simulink model "ArmDynamicsOnly"  (R2020a)
settings: Solver=FixedStepAuto  StartTime=0.0  StopTime=tsim  FixedStep=baseRate  MaxStep=0.0001  RelTol=1e-6  AbsTol=1e-6  EnableMultiTasking=on
values from neighbouring files (symbols this model uses):
  b0 = importdata("biases_layer_0.csv")    [Run_Initializer.m]
  b1 = importdata("biases_layer_1.csv")    [Run_Initializer.m]
  b_out = importdata("biases_output.csv")    [Run_Initializer.m]
  baseRate = 0.05    [Run_Initializer.m]
  CHASER_ABSOLUTE_POSITION = true    [Run_Initializer.m]
  drop_states_ARM = [ pi/2, pi/2, 0]    [Run_Initializer.m]
  drop_states_BLACK = [ xLength/2, yLength/2, pi]    [Run_Initializer.m]
  drop_states_BLUE = [ xLength/2, yLength/2, pi]    [Run_Initializer.m]
  drop_states_RED = [ xLength/2+0.5, yLength/2, pi]    [Run_Initializer.m]
  F_Black_X_nominal = 0.2196    [Run_Initializer.m]
  F_Black_Y_nominal = 0.2825    [Run_Initializer.m]
  F_Blue_X_nominal = 0.2196    [Run_Initializer.m]
  F_Blue_Y_nominal = 0.2825    [Run_Initializer.m]
  F_red_X_nominal = 0.2196    [Run_Initializer.m]
  F_red_Y_nominal = 0.2825    [Run_Initializer.m]
  F_thrusters_BLACK = [F_Black_X_nominal; F_Black_X_nominal;                             F_Black_Y_nominal; F_Black_Y_nominal; F_Black_X_nominal;                              F_Black_X_nominal; F_Black_Y_nominal; F_Black_Y_nominal]    [Run_Initializer.m]
  F_thrusters_BLUE = [F_Blue_X_nominal; F_Blue_X_nominal;                             F_Blue_Y_nominal; F_Blue_Y_nominal; F_Blue_X_nominal;                              F_Blue_X_nominal; F_Blue_Y_nominal; F_Blue_Y_nominal]    [Run_Initializer.m]
  F_thrusters_RED = [F_red_X_nominal; F_red_X_nominal;                             F_red_Y_nominal; F_red_Y_nominal; F_red_X_nominal;                              F_red_X_nominal; F_red_Y_nominal; F_red_Y_nominal]    [Run_Initializer.m]
  Gamma1_el = 0.12    [Run_Initializer.m]
  Gamma1_sh = 0.005    [Run_Initializer.m]
  Gamma1_wr = 0.025    [Run_Initializer.m]
  Gamma2_el = 5    [Run_Initializer.m]
  Gamma2_sh = 15    [Run_Initializer.m]
  Gamma2_wr = 5    [Run_Initializer.m]
  Gamma3_el = 10    [Run_Initializer.m]
  Gamma3_sh = 40    [Run_Initializer.m]
  Gamma3_wr = 40    [Run_Initializer.m]
  Gamma4_el = 0.039    [Run_Initializer.m]
  Gamma4_sh = 0.015    [Run_Initializer.m]
  Gamma4_wr = 0.029    [Run_Initializer.m]
  Gamma5_el = 800    [Run_Initializer.m]
  Gamma5_sh = 800    [Run_Initializer.m]
  Gamma5_wr = 800    [Run_Initializer.m]
  Gamma6_el = 0.000001    (= 1e-06)    [Run_Initializer.m]
  Gamma6_sh = 0.005    [Run_Initializer.m]
  Gamma6_wr = 0.02    [Run_Initializer.m]
  HOLD_POINT_RADIUS = 0.95    [Run_Initializer.m]
  home_states_BLACK = [ xLength/2; yLength/2; 0]    [Run_Initializer.m]
  home_states_BLUE = [ xLength/2; yLength/2; 0]    [Run_Initializer.m]
  home_states_RED = [ xLength/2+0.9; yLength/2; pi]    [Run_Initializer.m]
  init_states_BLACK = [ xLength/2; yLength/2; pi]    [Run_Initializer.m]
  init_states_BLUE = [ xLength/2; yLength/2; pi]    [Run_Initializer.m]
  init_states_RED = [ xLength/2+0.9; yLength/2; pi]    [Run_Initializer.m]
  Kd_tb = 1.0    (= 1)    [Run_Initializer.m]
  Kd_tblue = 1    [Run_Initializer.m]
  Kd_tr = 1.0    (= 1)    [Run_Initializer.m]
  Kd_xb = 8    [Run_Initializer.m]
  Kd_xblue = 8    [Run_Initializer.m]
  Kd_xr = 8    [Run_Initializer.m]
  Kd_yb = 8    [Run_Initializer.m]
  Kd_yblue = 8    [Run_Initializer.m]
  Kd_yr = 8    [Run_Initializer.m]
  Kp_tb = 0.1    [Run_Initializer.m]
  Kp_tblue = 0.1    [Run_Initializer.m]
  Kp_tr = 0.1    [Run_Initializer.m]
  Kp_xb = 2    [Run_Initializer.m]
  Kp_xblue = 2    [Run_Initializer.m]
  Kp_xr = 2    [Run_Initializer.m]
  Kp_yb = 2    [Run_Initializer.m]
  Kp_yblue = 2    [Run_Initializer.m]
  Kp_yr = 2    [Run_Initializer.m]
  MAX_BODY_ANGULAR_VELOCITY = 15*180/pi    (= 859.436692696)    [Run_Initializer.m]
  MAX_VELOCITY = 0.1    [Run_Initializer.m]
  noise_variance_BLACK = 0    [Run_Initializer.m]
  noise_variance_BLUE = 0    [Run_Initializer.m]
  noise_variance_RED = 0    [Run_Initializer.m]
  Phase0_End = Phase0_Duration    (= 10)    [Run_Initializer.m]
  Phase1_End = Phase0_Duration + Phase1_Duration    (= 15)    [Run_Initializer.m]
  Phase2_End = Phase0_Duration + Phase1_Duration +                                   Phase2_Duration    (= 45)    [Run_Initializer.m]
  Phase3_End = Phase0_Duration + Phase1_Duration +                                   Phase2_Duration + Phase3_Duration    (= 560)    [Run_Initializer.m]
  Phase3_SubPhase1_End = Phase2_End + Phase3_SubPhase1_Duration    (= 105)    [Run_Initializer.m]
  Phase3_SubPhase2_End = Phase2_End + Phase3_SubPhase1_Duration +                                   Phase3_SubPhase2_Duration    (= 210)    [Run_Initializer.m]
  Phase3_SubPhase3_End = Phase2_End + Phase3_SubPhase1_Duration +                                   Phase3_SubPhase2_Duration +                                  Phase3_SubPhase3_Duration    (= 240)    [Run_Initializer.m]
  Phase3_SubPhase4_End = Phase2_End + Phase3_SubPhase1_Duration +                                   Phase3_SubPhase2_Duration +                                  Phase3_SubPhase3_Duration +                                  Phase3_SubPhase4_Duration    [Run_Initializer.m]
  Phase4_End = Phase0_Duration + Phase1_Duration +                                   Phase2_Duration + Phase3_Duration +                                   Phase4_Duration    (= 680)    [Run_Initializer.m]
  Phase5_End = Phase0_Duration + Phase1_Duration +                                   Phase2_Duration + Phase3_Duration +                                   Phase4_Duration + Phase5_Duration    (= 700)    [Run_Initializer.m]
  relevant_half_range = (upper_state_bound - lower_state_bound)/2    [Run_Initializer.m]
  relevant_state_mean = (lower_state_bound + upper_state_bound)/2    [Run_Initializer.m]
  thruster_dist2CG_BLACK = [72.80;-65.20;61.75;-79.75;65.20;-65.20;74.25;-54.75]    [Run_Initializer.m]
  thruster_dist2CG_BLUE = [83.10;-54.90;71.50;-70.00;54.90;-75.50;64.50;-64.50]    [Run_Initializer.m]
  thruster_dist2CG_RED = [69.38;-56.62;50.01;-81.49;61.12;-68.38;78.99;-52.01]    [Run_Initializer.m]
  w0 = importdata("weights_layer_0.csv")    [Run_Initializer.m]
  w1 = importdata("weights_layer_1.csv")    [Run_Initializer.m]
  w_out = importdata("weights_output.csv")    [Run_Initializer.m]
  xLength = 3.51155    [Run_Initializer.m]
  yLength = 2.41935    [Run_Initializer.m]
undefined symbols (not defined in the file or in its folder): DiscIntNeverNeededParam, model_param, platformSelection, serverRate, simMode
libraries: dspstat3 x18, simulink x11, raspberrypiBasiclib x9, dspsigops x9, embdlinuxlib x7, MainLibrary x4, mspfiltlib x3, dsparch4 x3, etargetslib x1, sensehatlib x1
(part 1 of 14)
settings Model: ExtModeTrigDuration=2  Creator=AlexC  LastModifiedBy=alexa
settings SolverCC: PositivePriorityOrder=on
settings DataIOCC: ReturnWorkspaceOutputs=off
settings OptimizationCC: ZeroExternalMemoryAtStartup=off  ZeroInternalMemoryAtStartup=off  MaxStackSize=64
settings DebuggingCC: MultiTaskDSMMsg=none  ParameterTunabilityLossMsg=error  ArithmeticOperatorsInVariantConditions=warning
settings HardwareCC: ProdBitPerPointer=32  ProdBitPerSizeT=32  ProdBitPerPtrDiffT=32  ProdLargestAtomicInteger=Long  ProdLargestAtomicFloat=Double  ProdWordSize=32  ProdLongLongMode=on  ProdHWDeviceType=ARM Compatible->ARM Cortex
settings SFSimCC: CustomCodeUndefinedFunction=UseInterfaceOnly
settings RTWCC: SystemTargetFile=ert.tlc  HardwareBoard=Raspberry Pi  TemplateMakefile=ert_default_tmf  Toolchain=GNU GCC Raspberry Pi  BuildConfiguration=Faster Runs  TargetLang=C++
settings CodeAppCC: ForceParamTrailComments=on  OperatorAnnotations=on  StateflowObjectComments=on  MATLABSourceComments=on
settings ERTTargetCC: CodeReplacementLibrary=GCC ARM Cortex-A8  ERTCustomFileBanners=off  MatFileLogging=on  SupportContinuousTime=on  SupportNonInlinedSFcns=on  RemoveResetFunc=off  SupportVariableSizeSignals=on  ExtModeTransport=2  ExtModeStaticAlloc=on  ExtModeMexFile=ext_xcp  ExtModeIntrfLevel=Level2 - Open

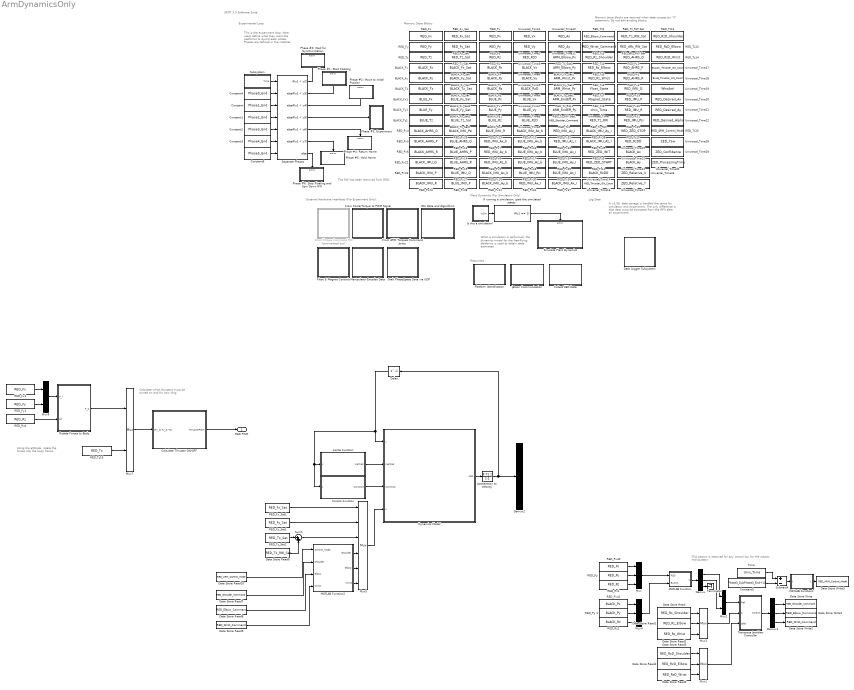
== system ArmDynamicsOnly ==
  note: This is the experiment loop; here, users define what they want the platforms to during each phase. Phases are defined in the intializer.
  note: External Hardware Interfaces (For Experiment Only):
  note: Resources
  note: Plant Dynamics (For Simulation Only)
  note: In v3.08, data storage is handled the same for simulation and experiment. The only difference is that data must be extracted from the RP3 after an experiment.
  note: When a simulation is performed, the dynamics model for the free-flying platforms is used to obtain state estimates.
  note: Memory Store Blocks
  note: SPOT 3.0
      | Software Suite
  note: Experimental Loop
  note: Log Data
  note: Memory store blocks are required when data crosses an "if" statement. Do not edit existing blocks.
  note: The RW has been removed from RED.
  note: This section is reserved for any control law for the robotic manipulator.
  note: Using the attitude, rotate the forces into the body frame.
  note: Calculate which thrusters must be turned on and for how long.
  Acceleration to Velocity : DiscreteIntegrator  IntegratorMethod=Integration: Backward Euler  InitialCondition=[drop_states_RED,drop_states_ARM,0,0,0,0,0,0]  SampleTime=-1  ICPrevOutput=DiscIntNeverNeededParam  ICPrevScaledInput=DiscIntNeverNeededParam
  BLACK_Fx : DataStoreMemory  DataStoreName=BLACK_Fx  ReadBeforeWriteMsg=warning  WriteAfterWriteMsg=warning  WriteAfterReadMsg=warning  ShowAdditionalParam=off
  BLACK_Fx1 : DataStoreMemory  DataStoreName=BLUE_Fx  ReadBeforeWriteMsg=warning  WriteAfterWriteMsg=warning  WriteAfterReadMsg=warning  ShowAdditionalParam=off
  BLACK_Fx_Sat : DataStoreMemory  DataStoreName=BLACK_Fx_Sat  ReadBeforeWriteMsg=warning  WriteAfterWriteMsg=warning  WriteAfterReadMsg=warning  ShowAdditionalParam=off
  BLACK_Fx_Sat1 : DataStoreMemory  DataStoreName=ARM_Elbow_Py  ReadBeforeWriteMsg=warning  WriteAfterWriteMsg=warning  WriteAfterReadMsg=warning  ShowAdditionalParam=off
  BLACK_Fx_Sat2 : DataStoreMemory  DataStoreName=BLUE_Fx_Sat  ReadBeforeWriteMsg=warning  WriteAfterWriteMsg=warning  WriteAfterReadMsg=warning  ShowAdditionalParam=off
  BLACK_Fy : DataStoreMemory  DataStoreName=BLACK_Fy  ReadBeforeWriteMsg=warning  WriteAfterWriteMsg=warning  WriteAfterReadMsg=warning  ShowAdditionalParam=off
  BLACK_Fy1 : DataStoreMemory  DataStoreName=BLUE_Fy  ReadBeforeWriteMsg=warning  WriteAfterWriteMsg=warning  WriteAfterReadMsg=warning  ShowAdditionalParam=off
  BLACK_Fy_Sat : DataStoreMemory  DataStoreName=BLACK_Fy_Sat  ReadBeforeWriteMsg=warning  WriteAfterWriteMsg=warning  WriteAfterReadMsg=warning  ShowAdditionalParam=off
  BLACK_Fy_Sat1 : DataStoreMemory  DataStoreName=ARM_Wrist_Px  ReadBeforeWriteMsg=warning  WriteAfterWriteMsg=warning  WriteAfterReadMsg=warning  ShowAdditionalParam=off
  BLACK_Fy_Sat2 : DataStoreMemory  DataStoreName=BLUE_Fy_Sat  ReadBeforeWriteMsg=warning  WriteAfterWriteMsg=warning  WriteAfterReadMsg=warning  ShowAdditionalParam=off
  BLACK_Px : DataStoreMemory  DataStoreName=BLACK_Px  ReadBeforeWriteMsg=warning  WriteAfterWriteMsg=warning  WriteAfterReadMsg=warning  ShowAdditionalParam=off
  BLACK_Px1 : DataStoreMemory  DataStoreName=BLUE_Px  ReadBeforeWriteMsg=warning  WriteAfterWriteMsg=warning  WriteAfterReadMsg=warning  ShowAdditionalParam=off
  BLACK_Py : DataStoreMemory  DataStoreName=BLACK_Py  ReadBeforeWriteMsg=warning  WriteAfterWriteMsg=warning  WriteAfterReadMsg=warning  ShowAdditionalParam=off
  BLACK_Py1 : DataStoreMemory  DataStoreName=BLUE_Py  ReadBeforeWriteMsg=warning  WriteAfterWriteMsg=warning  WriteAfterReadMsg=warning  ShowAdditionalParam=off
  BLACK_Rz : DataStoreMemory  DataStoreName=BLACK_Rz  ReadBeforeWriteMsg=warning  WriteAfterWriteMsg=warning  WriteAfterReadMsg=warning  ShowAdditionalParam=off
  BLACK_Rz1 : DataStoreMemory  DataStoreName=BLUE_Rz  ReadBeforeWriteMsg=warning  WriteAfterWriteMsg=warning  WriteAfterReadMsg=warning  ShowAdditionalParam=off
  BLACK_Tz : DataStoreMemory  DataStoreName=BLACK_Tz  ReadBeforeWriteMsg=warning  WriteAfterWriteMsg=warning  WriteAfterReadMsg=warning  ShowAdditionalParam=off
  BLACK_Tz1 : DataStoreMemory  DataStoreName=BLUE_Tz  ReadBeforeWriteMsg=warning  WriteAfterWriteMsg=warning  WriteAfterReadMsg=warning  ShowAdditionalParam=off
  BLACK_Tz_Sat : DataStoreMemory  DataStoreName=BLACK_Tz_Sat  ReadBeforeWriteMsg=warning  WriteAfterWriteMsg=warning  WriteAfterReadMsg=warning  ShowAdditionalParam=off
  BLACK_Tz_Sat1 : DataStoreMemory  DataStoreName=ARM_Wrist_Py  ReadBeforeWriteMsg=warning  WriteAfterWriteMsg=warning  WriteAfterReadMsg=warning  ShowAdditionalParam=off
  BLACK_Tz_Sat2 : DataStoreMemory  DataStoreName=BLUE_Tz_Sat  ReadBeforeWriteMsg=warning  WriteAfterWriteMsg=warning  WriteAfterReadMsg=warning  ShowAdditionalParam=off
  Calculate Thruster ON/OFF : Subsystem
  Collect ZED Data : Subsystem
  Constant : Constant  Value=Phase1_End  SampleTime=-1
  Constant1 : Constant  Value=Phase2_End  SampleTime=-1
  Constant2 : Constant  Value=Phase3_End  SampleTime=-1
  Constant3 : Constant  Value=Phase4_End  SampleTime=-1
  Constant4 : Constant  Value=Phase0_End  SampleTime=-1
  Constant5 : Constant  Value=Phase3_SubPhase3_End+10
  Constant6 : Constant  Value=Phase5_End  SampleTime=-1
  Coriolis Function : MATLAB Function  TreatAsAtomicUnit=on
  Data Logger Subsystem : Subsystem
  Data Store Read : DataStoreRead  DataStoreName=RED_Rz_Shoulder
  Data Store Read1 : DataStoreRead  DataStoreName=RED_Rz_Elbow
  Data Store Read10 : DataStoreRead  DataStoreName=RED_ARM_Control_Mode
  Data Store Read2 : DataStoreRead  DataStoreName=RED_Rz_Wrist
  Data Store Read3 : DataStoreRead  DataStoreName=RED_RzD_Shoulder
  Data Store Read4 : DataStoreRead  DataStoreName=RED_RzD_Elbow
  Data Store Read5 : DataStoreRead  DataStoreName=RED_RzD_Wrist
  Data Store Read6 : DataStoreRead  DataStoreName=RED_Tz_RW_Sat
  Data Store Read7 : DataStoreRead  DataStoreName=RED_Shoulder_Command
  Data Store Read8 : DataStoreRead  DataStoreName=RED_Elbow_Command
  Data Store Read9 : DataStoreRead  DataStoreName=RED_Wrist_Command
  Data Store Write : DataStoreWrite  DataStoreName=RED_Shoulder_Command
  Data Store Write1 : DataStoreWrite  DataStoreName=RED_Elbow_Command
  Data Store Write2 : DataStoreWrite  DataStoreName=RED_Wrist_Command
  Data Store Write3 : DataStoreWrite  DataStoreName=RED_ARM_Control_Mode
  Delay : Delay  DelayLength=1
  Demux : Demux  Outputs=3
  Demux1 : Demux  Outputs=3
  Demux2 : Demux  Outputs=12
  Dynamics Model : MATLAB Function  TreatAsAtomicUnit=on
  Float & Magnet Controls : Subsystem
  From ARM Torques Command Joints : Subsystem
  From Force/Torque to PWM Signal : Subsystem  SystemSampleTime=0.1
  From Torque Command RW : Subsystem  Commented=on
  Grab PhaseSpace Data via UDP : Subsystem
  IMU Data and Algorithms : Subsystem
  "If running a simulation, grab the simulated states." : If  IfExpression=u1 == 1  ShowElse=off
  "Inertia Function " : MATLAB Function  TreatAsAtomicUnit=on
  Is this a simulation? : Subsystem
  Jetson Communication : Subsystem
  MATLAB Function : MATLAB Function  TreatAsAtomicUnit=on
  MATLAB Function1 : MATLAB Function  TreatAsAtomicUnit=on
  MATLAB Function2 : MATLAB Function  TreatAsAtomicUnit=on
  Manipulator Encoder Data : Subsystem
  Mux{,1,3..4} (4 alike) : Mux  Inputs=3
  Mux2 : Mux  Inputs=2
  Mux5 : Mux  Inputs=6
  Mux6 : Mux  Inputs=2
  Mux7 : Mux  Inputs=2
  Phase #0: Wait for Synchronization : Subsystem  TreatAsAtomicUnit=on
  "Phase #1: Start Floating " : Subsystem  TreatAsAtomicUnit=on
  Phase #2: Move to Initial Position : Subsystem  TreatAsAtomicUnit=on
  Phase #3: Experiment : Subsystem  TreatAsAtomicUnit=on
  Phase #4: Return Home : Subsystem  TreatAsAtomicUnit=on
  Phase #5: Hold Home : Subsystem  TreatAsAtomicUnit=on
  Phase #6: Stop Floating and Spin Down RW : Subsystem  TreatAsAtomicUnit=on
  Platform Identification : Subsystem
  RED_Fx : DataStoreMemory  DataStoreName=RED_Fx  ReadBeforeWriteMsg=warning  WriteAfterWriteMsg=warning  WriteAfterReadMsg=warning  ShowAdditionalParam=off
  RED_Fx1 : DataStoreRead  DataStoreName=RED_Fx
  RED_Fx_Sat : DataStoreMemory  DataStoreName=RED_Fx_Sat  ReadBeforeWriteMsg=warning  WriteAfterWriteMsg=warning  WriteAfterReadMsg=warning  ShowAdditionalParam=off
  RED_Fx_Sat1 : DataStoreRead  DataStoreName=RED_Fx_Sat
  RED_Fy : DataStoreMemory  DataStoreName=RED_Fy  ReadBeforeWriteMsg=warning  WriteAfterWriteMsg=warning  WriteAfterReadMsg=warning  ShowAdditionalParam=off
  RED_Fy1 : DataStoreRead  DataStoreName=RED_Fy
  RED_Fy_Sat : DataStoreMemory  DataStoreName=RED_Fy_Sat  ReadBeforeWriteMsg=warning  WriteAfterWriteMsg=warning  WriteAfterReadMsg=warning  ShowAdditionalParam=off
  RED_Fy_Sat1 : DataStoreRead  DataStoreName=RED_Fy_Sat
  RED_Px : DataStoreMemory  DataStoreName=RED_Px  ReadBeforeWriteMsg=warning  WriteAfterWriteMsg=warning  WriteAfterReadMsg=warning  ShowAdditionalParam=off
  RED_Px1 : DataStoreMemory  DataStoreName=RED_AHRS_Q  ReadBeforeWriteMsg=warning  WriteAfterWriteMsg=warning  WriteAfterReadMsg=warning  ShowAdditionalParam=off
  RED_Px10 : DataStoreMemory  DataStoreName=BLACK_IMU_Ax_b  ReadBeforeWriteMsg=warning  WriteAfterWriteMsg=warning  WriteAfterReadMsg=warning  ShowAdditionalParam=off
  RED_Px11 : DataStoreMemory  DataStoreName=BLACK_IMU_Ay_b  ReadBeforeWriteMsg=warning  WriteAfterWriteMsg=warning  WriteAfterReadMsg=warning  ShowAdditionalParam=off
  RED_Px12 : DataStoreMemory  DataStoreName=BLACK_IMU_Az_b  ReadBeforeWriteMsg=warning  WriteAfterWriteMsg=warning  WriteAfterReadMsg=warning  ShowAdditionalParam=off
  RED_Px13 : DataStoreMemory  DataStoreName=BLUE_AHRS_Q  ReadBeforeWriteMsg=warning  WriteAfterWriteMsg=warning  WriteAfterReadMsg=warning  ShowAdditionalParam=off
  RED_Px14 : DataStoreMemory  DataStoreName=BLUE_AHRS_P  ReadBeforeWriteMsg=warning  WriteAfterWriteMsg=warning  WriteAfterReadMsg=warning  ShowAdditionalParam=off
  RED_Px15 : DataStoreMemory  DataStoreName=BLUE_AHRS_R  ReadBeforeWriteMsg=warning  WriteAfterWriteMsg=warning  WriteAfterReadMsg=warning  ShowAdditionalParam=off
  RED_Px16 : DataStoreMemory  DataStoreName=BLUE_IMU_Ax_b  ReadBeforeWriteMsg=warning  WriteAfterWriteMsg=warning  WriteAfterReadMsg=warning  ShowAdditionalParam=off
  RED_Px17 : DataStoreMemory  DataStoreName=BLUE_IMU_Ay_b  ReadBeforeWriteMsg=warning  WriteAfterWriteMsg=warning  WriteAfterReadMsg=warning  ShowAdditionalParam=off
  RED_Px18 : DataStoreMemory  DataStoreName=BLUE_IMU_Az_b  ReadBeforeWriteMsg=warning  WriteAfterWriteMsg=warning  WriteAfterReadMsg=warning  ShowAdditionalParam=off
  RED_Px19 : DataStoreMemory  DataStoreName=RED_IMU_Q  ReadBeforeWriteMsg=warning  WriteAfterWriteMsg=warning  WriteAfterReadMsg=warning  ShowAdditionalParam=off
  RED_Px2 : DataStoreMemory  DataStoreName=RED_AHRS_P  ReadBeforeWriteMsg=warning  WriteAfterWriteMsg=warning  WriteAfterReadMsg=warning  ShowAdditionalParam=off
  RED_Px20 : DataStoreMemory  DataStoreName=RED_IMU_P  ReadBeforeWriteMsg=warning  WriteAfterWriteMsg=warning  WriteAfterReadMsg=warning  ShowAdditionalParam=off
  RED_Px21 : DataStoreMemory  DataStoreName=RED_IMU_R  ReadBeforeWriteMsg=warning  WriteAfterWriteMsg=warning  WriteAfterReadMsg=warning  ShowAdditionalParam=off
  RED_Px22 : DataStoreMemory  DataStoreName=BLACK_IMU_Q  ReadBeforeWriteMsg=warning  WriteAfterWriteMsg=warning  WriteAfterReadMsg=warning  ShowAdditionalParam=off
  RED_Px23 : DataStoreMemory  DataStoreName=BLACK_IMU_P  ReadBeforeWriteMsg=warning  WriteAfterWriteMsg=warning  WriteAfterReadMsg=warning  ShowAdditionalParam=off
  RED_Px24 : DataStoreMemory  DataStoreName=BLACK_IMU_R  ReadBeforeWriteMsg=warning  WriteAfterWriteMsg=warning  WriteAfterReadMsg=warning  ShowAdditionalParam=off
  RED_Px25 : DataStoreMemory  DataStoreName=RED_IMU_Psi  ReadBeforeWriteMsg=warning  WriteAfterWriteMsg=warning  WriteAfterReadMsg=warning  ShowAdditionalParam=off
  RED_Px26 : DataStoreMemory  DataStoreName=BLACK_IMU_Psi  ReadBeforeWriteMsg=warning  WriteAfterWriteMsg=warning  WriteAfterReadMsg=warning  ShowAdditionalParam=off
  RED_Px27 : DataStoreMemory  DataStoreName=BLUE_IMU_Q  ReadBeforeWriteMsg=warning  WriteAfterWriteMsg=warning  WriteAfterReadMsg=warning  ShowAdditionalParam=off
  RED_Px28 : DataStoreMemory  DataStoreName=BLUE_IMU_P  ReadBeforeWriteMsg=warning  WriteAfterWriteMsg=warning  WriteAfterReadMsg=warning  ShowAdditionalParam=off
  RED_Px29 : DataStoreMemory  DataStoreName=BLUE_IMU_R  ReadBeforeWriteMsg=warning  WriteAfterWriteMsg=warning  WriteAfterReadMsg=warning  ShowAdditionalParam=off
  RED_Px3 : DataStoreMemory  DataStoreName=RED_AHRS_R  ReadBeforeWriteMsg=warning  WriteAfterWriteMsg=warning  WriteAfterReadMsg=warning  ShowAdditionalParam=off
  RED_Px30 : DataStoreMemory  DataStoreName=BLUE_IMU_Psi  ReadBeforeWriteMsg=warning  WriteAfterWriteMsg=warning  WriteAfterReadMsg=warning  ShowAdditionalParam=off
  RED_Px31 : DataStoreMemory  DataStoreName=RED_IMU_Ax_I  ReadBeforeWriteMsg=warning  WriteAfterWriteMsg=warning  WriteAfterReadMsg=warning  ShowAdditionalParam=off
  RED_Px32 : DataStoreMemory  DataStoreName=RED_IMU_Ay_I  ReadBeforeWriteMsg=warning  WriteAfterWriteMsg=warning  WriteAfterReadMsg=warning  ShowAdditionalParam=off
  RED_Px33 : DataStoreMemory  DataStoreName=RED_IMU_Az_I  ReadBeforeWriteMsg=warning  WriteAfterWriteMsg=warning  WriteAfterReadMsg=warning  ShowAdditionalParam=off
  RED_Px34 : DataStoreMemory  DataStoreName=BLUE_IMU_Ax_I  ReadBeforeWriteMsg=warning  WriteAfterWriteMsg=warning  WriteAfterReadMsg=warning  ShowAdditionalParam=off
  RED_Px35 : DataStoreMemory  DataStoreName=BLUE_IMU_Ay_I  ReadBeforeWriteMsg=warning  WriteAfterWriteMsg=warning  WriteAfterReadMsg=warning  ShowAdditionalParam=off
  RED_Px36 : DataStoreMemory  DataStoreName=BLUE_IMU_Az_I  ReadBeforeWriteMsg=warning  WriteAfterWriteMsg=warning  WriteAfterReadMsg=warning  ShowAdditionalParam=off
  RED_Px37 : DataStoreMemory  DataStoreName=BLACK_IMU_Ax_I  ReadBeforeWriteMsg=warning  WriteAfterWriteMsg=warning  WriteAfterReadMsg=warning  ShowAdditionalParam=off
  RED_Px38 : DataStoreMemory  DataStoreName=BLACK_IMU_Ay_I  ReadBeforeWriteMsg=warning  WriteAfterWriteMsg=warning  WriteAfterReadMsg=warning  ShowAdditionalParam=off
  RED_Px39 : DataStoreMemory  DataStoreName=BLACK_IMU_Az_I  ReadBeforeWriteMsg=warning  WriteAfterWriteMsg=warning  WriteAfterReadMsg=warning  ShowAdditionalParam=off
  RED_Px4 : DataStoreMemory  DataStoreName=BLACK_AHRS_Q  ReadBeforeWriteMsg=warning  WriteAfterWriteMsg=warning  WriteAfterReadMsg=warning  ShowAdditionalParam=off
  RED_Px40 : DataStoreRead  DataStoreName=RED_Px
  RED_Px41 : DataStoreRead  DataStoreName=BLACK_Px
  RED_Px5 : DataStoreMemory  DataStoreName=BLACK_AHRS_P  ReadBeforeWriteMsg=warning  WriteAfterWriteMsg=warning  WriteAfterReadMsg=warning  ShowAdditionalParam=off
  RED_Px6 : DataStoreMemory  DataStoreName=BLACK_AHRS_R  ReadBeforeWriteMsg=warning  WriteAfterWriteMsg=warning  WriteAfterReadMsg=warning  ShowAdditionalParam=off
  RED_Px7 : DataStoreMemory  DataStoreName=RED_IMU_Ax_b  ReadBeforeWriteMsg=warning  WriteAfterWriteMsg=warning  WriteAfterReadMsg=warning  ShowAdditionalParam=off
  RED_Px8 : DataStoreMemory  DataStoreName=RED_IMU_Ay_b  ReadBeforeWriteMsg=warning  WriteAfterWriteMsg=warning  WriteAfterReadMsg=warning  ShowAdditionalParam=off
  RED_Px9 : DataStoreMemory  DataStoreName=RED_IMU_Az_b  ReadBeforeWriteMsg=warning  WriteAfterWriteMsg=warning  WriteAfterReadMsg=warning  ShowAdditionalParam=off
  RED_Py : DataStoreMemory  DataStoreName=RED_Py  ReadBeforeWriteMsg=warning  WriteAfterWriteMsg=warning  WriteAfterReadMsg=warning  ShowAdditionalParam=off
  "RED_Py " : DataStoreRead  DataStoreName=RED_Py
  RED_Py 1 : DataStoreRead  DataStoreName=BLACK_Py
  RED_Rz : DataStoreMemory  DataStoreName=RED_Rz  ReadBeforeWriteMsg=warning  WriteAfterWriteMsg=warning  WriteAfterReadMsg=warning  ShowAdditionalParam=off
  RED_Rz1 : DataStoreRead  DataStoreName=RED_Rz
  RED_Rz2 : DataStoreRead  DataStoreName=BLACK_Rz
  RED_Rz4 : DataStoreRead  DataStoreName=RED_Rz
  RED_Tz : DataStoreMemory  DataStoreName=RED_Tz  ReadBeforeWriteMsg=warning  WriteAfterWriteMsg=warning  WriteAfterReadMsg=warning  ShowAdditionalParam=off
  RED_Tz1 : DataStoreMemory  DataStoreName=RED_Shoulder_Command  ReadBeforeWriteMsg=warning  WriteAfterWriteMsg=warning  WriteAfterReadMsg=warning  ShowAdditionalParam=off
  RED_Tz10 : DataStoreMemory  DataStoreName=RED_ZED_STOP  ReadBeforeWriteMsg=warning  WriteAfterWriteMsg=warning  WriteAfterReadMsg=warning  ShowAdditionalParam=off
  RED_Tz11 : DataStoreMemory  DataStoreName=RED_ZED_START  ReadBeforeWriteMsg=warning  WriteAfterWriteMsg=warning  WriteAfterReadMsg=warning  ShowAdditionalParam=off
  RED_Tz12 : DataStoreMemory  DataStoreName=RED_RzD_Shoulder  ReadBeforeWriteMsg=warning  WriteAfterWriteMsg=warning  WriteAfterReadMsg=warning  ShowAdditionalParam=off
  RED_Tz13 : DataStoreMemory  DataStoreName=RED_RzD_Elbow  ReadBeforeWriteMsg=warning  WriteAfterWriteMsg=warning  WriteAfterReadMsg=warning  ShowAdditionalParam=off
  RED_Tz14 : DataStoreMemory  DataStoreName=RED_RzD_Wrist  ReadBeforeWriteMsg=warning  WriteAfterWriteMsg=warning  WriteAfterReadMsg=warning  ShowAdditionalParam=off
  RED_Tz15 : DataStoreMemory  DataStoreName=RED_ARM_Control_Mode  ReadBeforeWriteMsg=warning  WriteAfterWriteMsg=warning  WriteAfterReadMsg=warning  ShowAdditionalParam=off
  RED_Tz16 : DataStoreRead  DataStoreName=RED_Tz
  RED_Tz2 : DataStoreMemory  DataStoreName=RED_Elbow_Command  ReadBeforeWriteMsg=warning  WriteAfterWriteMsg=warning  WriteAfterReadMsg=warning  ShowAdditionalParam=off
  RED_Tz3 : DataStoreMemory  DataStoreName=RED_Wrist_Command  ReadBeforeWriteMsg=warning  WriteAfterWriteMsg=warning  WriteAfterReadMsg=warning  ShowAdditionalParam=off
  RED_Tz4 : DataStoreMemory  DataStoreName=RED_Rz_Shoulder  ReadBeforeWriteMsg=warning  WriteAfterWriteMsg=warning  WriteAfterReadMsg=warning  ShowAdditionalParam=off
  RED_Tz5 : DataStoreMemory  DataStoreName=RED_Rz_Elbow  ReadBeforeWriteMsg=warning  WriteAfterWriteMsg=warning  WriteAfterReadMsg=warning  ShowAdditionalParam=off
  RED_Tz6 : DataStoreMemory  DataStoreName=RED_Rz_Wrist  ReadBeforeWriteMsg=warning  WriteAfterWriteMsg=warning  WriteAfterReadMsg=warning  ShowAdditionalParam=off
  RED_Tz7 : DataStoreMemory  DataStoreName=Float_State  ReadBeforeWriteMsg=warning  WriteAfterWriteMsg=warning  WriteAfterReadMsg=warning  ShowAdditionalParam=off
  RED_Tz8 : DataStoreMemory  DataStoreName=Magnet_State  ReadBeforeWriteMsg=warning  WriteAfterWriteMsg=warning  WriteAfterReadMsg=warning  ShowAdditionalParam=off
  RED_Tz9 : DataStoreMemory  DataStoreName=RED_ZED_INIT  ReadBeforeWriteMsg=warning  WriteAfterWriteMsg=warning  WriteAfterReadMsg=warning  ShowAdditionalParam=off
  RED_Tz_RW : DataStoreMemory  DataStoreName=RED_Tz_RW  ReadBeforeWriteMsg=warning  WriteAfterWriteMsg=warning  WriteAfterReadMsg=warning  ShowAdditionalParam=off
  RED_Tz_RW Sat : DataStoreMemory  DataStoreName=RED_Tz_RW_Sat  ReadBeforeWriteMsg=warning  WriteAfterWriteMsg=warning  WriteAfterReadMsg=warning  ShowAdditionalParam=off
  RED_Tz_RW Sat1 : DataStoreMemory  DataStoreName=ARM_EndEff_Py  ReadBeforeWriteMsg=warning  WriteAfterWriteMsg=warning  WriteAfterReadMsg=warning  ShowAdditionalParam=off
  RED_Tz_RW1 : DataStoreMemory  DataStoreName=ARM_EndEff_Px  ReadBeforeWriteMsg=warning  WriteAfterWriteMsg=warning  WriteAfterReadMsg=warning  ShowAdditionalParam=off
  RED_Tz_Sat : DataStoreMemory  DataStoreName=RED_Tz_Sat  ReadBeforeWriteMsg=warning  WriteAfterWriteMsg=warning  WriteAfterReadMsg=warning  ShowAdditionalParam=off
  RED_Tz_Sat1 : DataStoreMemory  DataStoreName=ARM_Elbow_Px  ReadBeforeWriteMsg=warning  WriteAfterWriteMsg=warning  WriteAfterReadMsg=warning  ShowAdditionalParam=off
  RED_Tz_Sat2 : DataStoreRead  DataStoreName=RED_Tz_Sat
  RED_dRz_RW Sat : DataStoreMemory  DataStoreName=RED_dRz_RW_Sat  ReadBeforeWriteMsg=warning  WriteAfterWriteMsg=warning  WriteAfterReadMsg=warning  ShowAdditionalParam=off
  Rotate Forces to Body : Subsystem
  Separate Phases : If  NumInputs=7  IfExpression=u1 < u2  ElseIfExpressions=u1 < u3, u1 < u4, u1 < u5, u1 < u6, u1 < u7
  Simulate Plant Dynamics : Subsystem  TreatAsAtomicUnit=on
  Subsystem : Subsystem
  Subtract4 : Sum  Inputs=+-
  Sum1 : Sum  Inputs=|++
  Terminator : Terminator
  Time : DataStoreRead  DataStoreName=Univ_Time
  Transpose Jacobian Controller : Subsystem
  Universal_Time : DataStoreMemory  DataStoreName=Univ_Time  ReadBeforeWriteMsg=warning  WriteAfterWriteMsg=warning  WriteAfterReadMsg=warning  ShowAdditionalParam=off
  Universal_Time1 : DataStoreMemory  DataStoreName=RED_Vx  ReadBeforeWriteMsg=warning  WriteAfterWriteMsg=warning  WriteAfterReadMsg=warning  ShowAdditionalParam=off
  Universal_Time10 : DataStoreMemory  DataStoreName=RED_Ax  ReadBeforeWriteMsg=warning  WriteAfterWriteMsg=warning  WriteAfterReadMsg=warning  ShowAdditionalParam=off
  Universal_Time11 : DataStoreMemory  DataStoreName=RED_Ay  ReadBeforeWriteMsg=warning  WriteAfterWriteMsg=warning  WriteAfterReadMsg=warning  ShowAdditionalParam=off
  Universal_Time12 : DataStoreMemory  DataStoreName=BLACK_Ax  ReadBeforeWriteMsg=warning  WriteAfterWriteMsg=warning  WriteAfterReadMsg=warning  ShowAdditionalParam=off
  Universal_Time13 : DataStoreMemory  DataStoreName=BLACK_Ay  ReadBeforeWriteMsg=warning  WriteAfterWriteMsg=warning  WriteAfterReadMsg=warning  ShowAdditionalParam=off
  Universal_Time14 : DataStoreMemory  DataStoreName=BLACK_RzDD  ReadBeforeWriteMsg=warning  WriteAfterWriteMsg=warning  WriteAfterReadMsg=warning  ShowAdditionalParam=off
  Universal_Time15 : DataStoreMemory  DataStoreName=RED_RzDD  ReadBeforeWriteMsg=warning  WriteAfterWriteMsg=warning  WriteAfterReadMsg=warning  ShowAdditionalParam=off
  Universal_Time16 : DataStoreMemory  DataStoreName=RED_Thruster_ON_Count  ReadBeforeWriteMsg=warning  WriteAfterWriteMsg=warning  WriteAfterReadMsg=warning  ShowAdditionalParam=off
  Universal_Time17 : DataStoreMemory  DataStoreName=BLACK_Thruster_ON_Count  ReadBeforeWriteMsg=warning  WriteAfterWriteMsg=warning  WriteAfterReadMsg=warning  ShowAdditionalParam=off
  Universal_Time18 : DataStoreMemory  DataStoreName=BLUE_Thruster_ON_Count  ReadBeforeWriteMsg=warning  WriteAfterWriteMsg=warning  WriteAfterReadMsg=warning  ShowAdditionalParam=off
  Universal_Time19 : DataStoreMemory  DataStoreName=WhoAmI  ReadBeforeWriteMsg=warning  WriteAfterWriteMsg=warning  WriteAfterReadMsg=warning  ShowAdditionalParam=off
  Universal_Time2 : DataStoreMemory  DataStoreName=RED_Vy  ReadBeforeWriteMsg=warning  WriteAfterWriteMsg=warning  WriteAfterReadMsg=warning  ShowAdditionalParam=off
  Universal_Time20 : DataStoreMemory  DataStoreName=RED_Desired_Ax  ReadBeforeWriteMsg=warning  WriteAfterWriteMsg=warning  WriteAfterReadMsg=warning  ShowAdditionalParam=off
  Universal_Time21 : DataStoreMemory  DataStoreName=RED_Desired_Ay  ReadBeforeWriteMsg=warning  WriteAfterWriteMsg=warning  WriteAfterReadMsg=warning  ShowAdditionalParam=off
  Universal_Time22 : DataStoreMemory  DataStoreName=RED_Desired_Alpha  ReadBeforeWriteMsg=warning  WriteAfterWriteMsg=warning  WriteAfterReadMsg=warning  ShowAdditionalParam=off
  Universal_Time26 : DataStoreMemory  DataStoreName=ZED_Relative_X  ReadBeforeWriteMsg=warning  WriteAfterWriteMsg=warning  WriteAfterReadMsg=warning  ShowAdditionalParam=off
  Universal_Time27 : DataStoreMemory  DataStoreName=ZED_Relative_Y  ReadBeforeWriteMsg=warning  WriteAfterWriteMsg=warning  WriteAfterReadMsg=warning  ShowAdditionalParam=off
  Universal_Time28 : DataStoreMemory  DataStoreName=ZED_Yaw  ReadBeforeWriteMsg=warning  WriteAfterWriteMsg=warning  WriteAfterReadMsg=warning  ShowAdditionalParam=off
  Universal_Time29 : DataStoreMemory  DataStoreName=ZED_Confidence  ReadBeforeWriteMsg=warning  WriteAfterWriteMsg=warning  WriteAfterReadMsg=warning  ShowAdditionalParam=off
  Universal_Time3 : DataStoreMemory  DataStoreName=RED_RzD  ReadBeforeWriteMsg=warning  WriteAfterWriteMsg=warning  WriteAfterReadMsg=warning  ShowAdditionalParam=off
  Universal_Time30 : DataStoreMemory  DataStoreName=ZED_ProcessingTime  ReadBeforeWriteMsg=warning  WriteAfterWriteMsg=warning  WriteAfterReadMsg=warning  ShowAdditionalParam=off
  Universal_Time4 : DataStoreMemory  DataStoreName=BLACK_Vx  ReadBeforeWriteMsg=warning  WriteAfterWriteMsg=warning  WriteAfterReadMsg=warning  ShowAdditionalParam=off
  Universal_Time5 : DataStoreMemory  DataStoreName=BLACK_Vy  ReadBeforeWriteMsg=warning  WriteAfterWriteMsg=warning  WriteAfterReadMsg=warning  ShowAdditionalParam=off
  Universal_Time6 : DataStoreMemory  DataStoreName=BLACK_RzD  ReadBeforeWriteMsg=warning  WriteAfterWriteMsg=warning  WriteAfterReadMsg=warning  ShowAdditionalParam=off
  Universal_Time7 : DataStoreMemory  DataStoreName=BLUE_Vx  ReadBeforeWriteMsg=warning  WriteAfterWriteMsg=warning  WriteAfterReadMsg=warning  ShowAdditionalParam=off
  Universal_Time8 : DataStoreMemory  DataStoreName=BLUE_Vy  ReadBeforeWriteMsg=warning  WriteAfterWriteMsg=warning  WriteAfterReadMsg=warning  ShowAdditionalParam=off
  Universal_Time9 : DataStoreMemory  DataStoreName=BLUE_RzD  ReadBeforeWriteMsg=warning  WriteAfterWriteMsg=warning  WriteAfterReadMsg=warning  ShowAdditionalParam=off
  RED PWM : Outport  VectorParamsAs1DForOutWhenUnconnected=off
  wires:
  "If running a simulation, grab the simulated states."/1 -> Simulate Plant Dynamics/Action
  Separate Phases/3 -> Phase #2: Move to Initial Position/Action
  Constant1/1 -> Separate Phases/4
  Constant/1 -> Separate Phases/3
  Subsystem/1(Time) -> Separate Phases/1
  Separate Phases/1 -> Phase #0: Wait for Synchronization/Action
  Is this a simulation?/1(isSim) -> "If running a simulation, grab the simulated states."/1
  Constant2/1 -> Separate Phases/5
  Separate Phases/2 -> "Phase #1: Start Floating "/Action
  Separate Phases/6 -> Phase #5: Hold Home/Action
  Separate Phases/5 -> Phase #4: Return Home/Action
  Separate Phases/4 -> Phase #3: Experiment/Action
  Separate Phases/7 -> Phase #6: Stop Floating and Spin Down RW/Action
  Constant6/1 -> Separate Phases/7
  Constant4/1 -> Separate Phases/2
  Constant3/1 -> Separate Phases/6
  Demux/1 -> Mux2/1
  Mux/1 -> MATLAB Function/1(RED)
  RED_Px41/1 -> Mux4/1
  Mux2/1 -> Transpose Jacobian Controller/1(Ref)
  Subtract4/1 -> MATLAB Function1/1(Sim_Time)
  Mux4/1 -> MATLAB Function/2(BLACK)
  "RED_Py "/1 -> Mux/2
  Time/1 -> Subtract4/1
  Constant5/1 -> Subtract4/2
  Data Store Read5/1 -> Mux1/3
  RED_Py 1/1 -> Mux4/2
  RED_Rz1/1 -> Mux/3
  Demux/3 -> Terminator/1
  Mux1/1 -> Transpose Jacobian Controller/3(qdot)
  Data Store Read3/1 -> Mux1/1
  Mux3/1 -> Transpose Jacobian Controller/2(q)
  RED_Rz2/1 -> Mux4/3
  Data Store Read2/1 -> Mux3/3
  Demux1/2 -> Data Store Write1/1
  Data Store Read/1 -> Mux3/1
  Transpose Jacobian Controller/1(Control) -> Demux1/1
  Demux1/3 -> Data Store Write2/1
  Data Store Read1/1 -> Mux3/2
  MATLAB Function/1(p_red_target) -> Demux/1
  MATLAB Function1/1(Control_Mode) -> Data Store Write3/1
  Data Store Read4/1 -> Mux1/2
  Demux1/1 -> Data Store Write/1
  RED_Px40/1 -> Mux/1
  Demux/2 -> Mux2/2
  Data Store Read8/1 -> MATLAB Function2/3("Elbow ")
  Data Store Read9/1 -> MATLAB Function2/4("Wrist ")
  Data Store Read10/1 -> MATLAB Function2/1(Control_Mode)
  Coriolis Function/1(CoriolisS) -> Dynamics Model/3(CoriolisS)
  RED_Fy_Sat1/1 -> Mux5/2
  Dynamics Model/1(xdot) -> Acceleration to Velocity/1
  "Inertia Function "/1(InertiaS) -> Dynamics Model/2(InertiaS)
  Acceleration to Velocity/1 -> Delay/1, Demux2/1
  MATLAB Function2/1(Shoulder) -> Mux5/4
  MATLAB Function2/2(Elbow) -> Mux5/5
  Data Store Read6/1 -> Sum1/2
  MATLAB Function2/3(Wrist) -> Mux5/6
  Data Store Read7/1 -> MATLAB Function2/2("Shoulder ")
  RED_Fx_Sat1/1 -> Mux5/1
  Sum1/1 -> Mux5/3
  Delay/1 -> Coriolis Function/1(x), "Inertia Function "/1(x), Dynamics Model/1(x)
  RED_Tz_Sat2/1 -> Sum1/1
  Mux5/1 -> Dynamics Model/4(u)
  Calculate Thruster ON/OFF/1(ThrusterPWM) -> RED PWM/1
  Rotate Forces to Body/1(F_b) -> Mux7/1
  RED_Fx1/1 -> Mux6/1
  Mux7/1 -> Calculate Thruster ON/OFF/1("[Fx_b; Fy_b; Tz]")
  RED_Tz16/1 -> Mux7/2
  RED_Fy1/1 -> Mux6/2
  RED_Rz4/1 -> Rotate Forces to Body/2(Rz)
  Mux6/1 -> Rotate Forces to Body/1("F_I ")

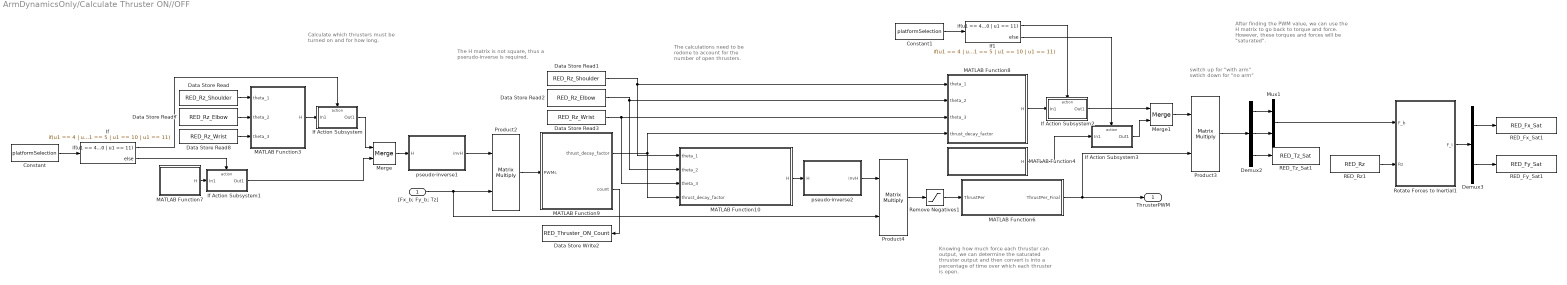
== system ArmDynamicsOnly/Calculate Thruster ON//OFF ==
  note: switch up for "with arm"
      | swtich down for "no arm"
  note: Knowing how much force each thruster can output, we can determine the saturated thruster output and then convert is into a percentage of time over which each thruster is open.
  note: The H matrix is not square, thus a pserudo-inverse is required.
  note: After finding the PWM value, we can use the H matrix to go back to torque and force. However, these torques and forces will be "saturated".
  note: Calculate which thrusters must be turned on and for how long.
  note: The calculations need to be redone to account for the number of open thrusters.
  "[Fx_b; Fy_b; Tz]" : Inport
  Constant : Constant  Value=platformSelection
  Constant1 : Constant  Value=platformSelection
  Data Store Read : DataStoreRead  DataStoreName=RED_Rz_Shoulder
  Data Store Read1 : DataStoreRead  DataStoreName=RED_Rz_Shoulder
  Data Store Read2 : DataStoreRead  DataStoreName=RED_Rz_Elbow
  Data Store Read3 : DataStoreRead  DataStoreName=RED_Rz_Wrist
  Data Store Read7 : DataStoreRead  DataStoreName=RED_Rz_Elbow
  Data Store Read8 : DataStoreRead  DataStoreName=RED_Rz_Wrist
  Data Store Write2 : DataStoreWrite  DataStoreName=RED_Thruster_ON_Count
  Demux2 : Demux  Outputs=3
  Demux3 : Demux  Outputs=2
  If : If  IfExpression=u1 == 4 | u1 == 5 | u1 == 10 | u1 == 11
  If Action Subsystem : Subsystem  TreatAsAtomicUnit=on
  If Action Subsystem1 : Subsystem  TreatAsAtomicUnit=on
  If Action Subsystem2 : Subsystem  TreatAsAtomicUnit=on
  If Action Subsystem3 : Subsystem  TreatAsAtomicUnit=on
  If1 : If  IfExpression=u1 == 4 | u1 == 5 | u1 == 10 | u1 == 11
  MATLAB Function10 : MATLAB Function  TreatAsAtomicUnit=on
  MATLAB Function3 : MATLAB Function  TreatAsAtomicUnit=on
  MATLAB Function4 : MATLAB Function  TreatAsAtomicUnit=on
  MATLAB Function6 : MATLAB Function  TreatAsAtomicUnit=on
  MATLAB Function7 : MATLAB Function  TreatAsAtomicUnit=on
  MATLAB Function8 : MATLAB Function  TreatAsAtomicUnit=on
  MATLAB Function9 : MATLAB Function  TreatAsAtomicUnit=on
  Merge : Merge
  Merge1 : Merge
  Mux1 : Mux  Inputs=2
  Product2 : Product  Multiplication=Matrix(*)
  Product3 : Product  Multiplication=Matrix(*)
  Product4 : Product  Multiplication=Matrix(*)
  RED_Fx_Sat1 : DataStoreWrite  DataStoreName=RED_Fx_Sat
  RED_Fy_Sat1 : DataStoreWrite  DataStoreName=RED_Fy_Sat
  RED_Rz1 : DataStoreRead  DataStoreName=RED_Rz
  RED_Tz_Sat1 : DataStoreWrite  DataStoreName=RED_Tz_Sat
  Remove Negatives1 : Saturate  UpperLimit=1000  LowerLimit=0
  Rotate Forces to Inertial1 : Subsystem
  pseudo-inverse1 : Subsystem
  pseudo-inverse2 : Subsystem
  ThrusterPWM : Outport  VectorParamsAs1DForOutWhenUnconnected=off
  wires:
  MATLAB Function7/1(H) -> If Action Subsystem1/1(In1)
  If Action Subsystem3/1(Out1) -> Merge1/2
  Demux2/3 -> RED_Tz_Sat1/1
  Product3/1 -> Demux2/1
  Data Store Read8/1 -> MATLAB Function3/3(theta_3)
  Data Store Read2/1 -> MATLAB Function8/2(theta_2), MATLAB Function10/2(theta_2)
  MATLAB Function8/1(H) -> If Action Subsystem2/1(In1)
  Data Store Read/1 -> MATLAB Function3/1(theta_1)
  If1/2 -> If Action Subsystem3/Action
  Demux3/2 -> RED_Fy_Sat1/1
  MATLAB Function9/2(count) -> Data Store Write2/1
  If Action Subsystem/1(Out1) -> Merge/1
  MATLAB Function3/1(H) -> If Action Subsystem/1(In1)
  RED_Rz1/1 -> Rotate Forces to Inertial1/2(Rz)
  Data Store Read3/1 -> MATLAB Function8/3(theta_3), MATLAB Function10/3(theta_3)
  MATLAB Function4/1(H) -> If Action Subsystem3/1(In1)
  Demux3/1 -> RED_Fx_Sat1/1
  pseudo-inverse1/1(invH) -> Product2/1
  MATLAB Function6/1(ThrustPer_Final) -> ThrusterPWM/1, Product3/2
  If Action Subsystem1/1(Out1) -> Merge/2
  Demux2/2 -> Mux1/2
  Constant1/1 -> If1/1
  If Action Subsystem2/1(Out1) -> Merge1/1
  Demux2/1 -> Mux1/1
  "[Fx_b; Fy_b; Tz]"/1 -> Product4/2, Product2/2
  MATLAB Function9/1(thrust_decay_factor) -> MATLAB Function10/4(thrust_decay_factor), MATLAB Function8/4(thrust_decay_factor)
  If/2 -> If Action Subsystem1/Action
  Mux1/1 -> Rotate Forces to Inertial1/1("F_b ")
  Product2/1 -> MATLAB Function9/1(PWMs)
  Product4/1 -> Remove Negatives1/1
  Rotate Forces to Inertial1/1(F_I) -> Demux3/1
  If/1 -> If Action Subsystem/Action
  Remove Negatives1/1 -> MATLAB Function6/1(ThrustPer)
  MATLAB Function10/1(H) -> pseudo-inverse2/1(H)
  If1/1 -> If Action Subsystem2/Action
  Data Store Read7/1 -> MATLAB Function3/2(theta_2)
  Constant/1 -> If/1
  Merge/1 -> pseudo-inverse1/1(H)
  Data Store Read1/1 -> MATLAB Function8/1(theta_1), MATLAB Function10/1(theta_1)
  Merge1/1 -> Product3/1
  pseudo-inverse2/1(invH) -> Product4/1

== system ArmDynamicsOnly/Collect ZED Data ==
  Byte Unpack : etargetslib/Byte Unpack  dimensions={[1],[1],[1],[1],[1]}  datatypes={'single','single','single','single','single'}  byteAlign=1
  Data Store Write : DataStoreWrite  DataStoreName=ZED_Relative_X
  Data Store Write1 : DataStoreWrite  DataStoreName=ZED_Relative_Y
  Data Store Write2 : DataStoreWrite  DataStoreName=ZED_Yaw
  Data Store Write3 : DataStoreWrite  DataStoreName=ZED_Confidence
  Data Store Write7 : DataStoreWrite  DataStoreName=ZED_ProcessingTime
  Data Type Conversion{,1..4} (5 alike) : DataTypeConversion  OutDataTypeStr=double
  Terminator1 : Terminator
  UDP Receive : embdlinuxlib/UDP Receive  localURL='0.0.0.0'  localPort=30172  remoteURL='0.0.0.0'  remotePort=-1  recvBufferSize=8192  signalDatatype=uint8  dims=20  isVarSize=off  showBlockingTime=off  blockingTime=0  sampletime=0.05  blockPlatform=Raspberry Pi
      settings: SourceProductBaseCode=SC_BEAGLEBONE_BLUE,RASPPI
  wires:
  Byte Unpack/4 -> Data Type Conversion3/1
  Data Type Conversion/1 -> Data Store Write/1
  UDP Receive/2 -> Terminator1/1
  Data Type Conversion1/1 -> Data Store Write1/1
  Data Type Conversion3/1 -> Data Store Write3/1
  Byte Unpack/5 -> Data Type Conversion4/1
  Byte Unpack/1 -> Data Type Conversion/1
  UDP Receive/1 -> Byte Unpack/1
  Data Type Conversion2/1 -> Data Store Write2/1
  Byte Unpack/3 -> Data Type Conversion2/1
  Data Type Conversion4/1 -> Data Store Write7/1
  Byte Unpack/2 -> Data Type Conversion1/1
